simulink model "CommandGenerator"  (R2025b)
settings: Solver=FixedStepDiscrete  StartTime=0.0  StopTime=10  FixedStep=double(CMD_SAMPLE_TIME)  RelTol=1e-3
values from neighbouring files (symbols this model uses):
  CMD_HOVER_POS_NED : value not decoded    [CommandDict.sldd]
  CMD_HOVER_VALID = 1    [CommandDict.sldd]
  CMD_HOVER_VEL_NED : value not decoded    [CommandDict.sldd]
  CMD_HOVER_YAW = 0.0    [CommandDict.sldd]
  CMD_MODE_POS_HOLD = 1    [CommandDict.sldd]
  CMD_SAMPLE_TIME = 0.001    [CommandDict.sldd]
settings Model: DataDictionary=CommandDict.sldd  Creator=89447  LastModifiedBy=89447

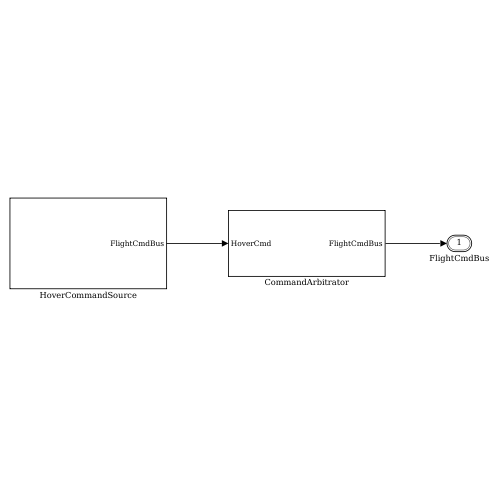
[thumbnail: Simulink's stored preview of the top-level diagram]
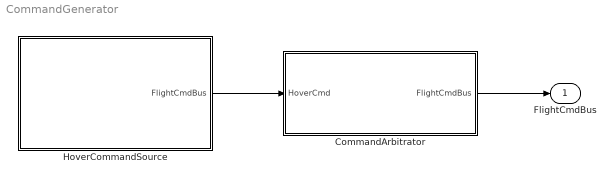
== system CommandGenerator ==
  CommandArbitrator : Subsystem
  HoverCommandSource : Subsystem
  FlightCmdBus : Outport  OutDataTypeStr=Bus: FlightCmdBus
  wires:
  HoverCommandSource/1(FlightCmdBus) -> CommandArbitrator/1(HoverCmd)
  CommandArbitrator/1(FlightCmdBus) -> FlightCmdBus/1

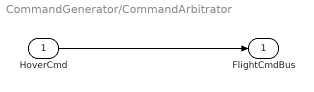
== system CommandGenerator/CommandArbitrator ==
  HoverCmd : Inport  OutDataTypeStr=Bus: FlightCmdBus
  FlightCmdBus : Outport  OutDataTypeStr=Bus: FlightCmdBus
  wires:
  HoverCmd/1 -> FlightCmdBus/1

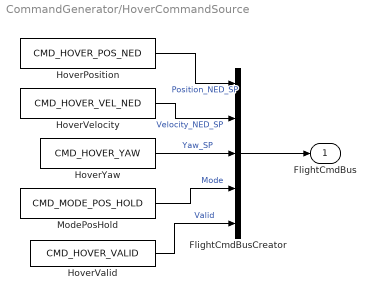
== system CommandGenerator/HoverCommandSource ==
  FlightCmdBusCreator : BusCreator  Inputs=5  OutDataTypeStr=Bus: FlightCmdBus  NonVirtualBus=on
  HoverPosition : Constant  Value=CMD_HOVER_POS_NED  OutDataTypeStr=single  SampleTime=double(CMD_SAMPLE_TIME)
  HoverValid : Constant  Value=CMD_HOVER_VALID  OutDataTypeStr=boolean  SampleTime=double(CMD_SAMPLE_TIME)
  HoverVelocity : Constant  Value=CMD_HOVER_VEL_NED  OutDataTypeStr=single  SampleTime=double(CMD_SAMPLE_TIME)
  HoverYaw : Constant  Value=CMD_HOVER_YAW  OutDataTypeStr=single  SampleTime=double(CMD_SAMPLE_TIME)
  ModePosHold : Constant  Value=CMD_MODE_POS_HOLD  OutDataTypeStr=uint8  SampleTime=double(CMD_SAMPLE_TIME)
  FlightCmdBus : Outport  OutDataTypeStr=Bus: FlightCmdBus
  wires:
  HoverPosition/1 -> FlightCmdBusCreator/1  "Position_NED_SP"
  HoverVelocity/1 -> FlightCmdBusCreator/2  "Velocity_NED_SP"
  HoverYaw/1 -> FlightCmdBusCreator/3  "Yaw_SP"
  ModePosHold/1 -> FlightCmdBusCreator/4  "Mode"
  HoverValid/1 -> FlightCmdBusCreator/5  "Valid"
  FlightCmdBusCreator/1 -> FlightCmdBus/1
